simulink model "Watermarker"  (R2022a)
settings: Solver=FixedStepDiscrete  StartTime=0.0  StopTime=256*256-1  RelTol=1e-3
values from neighbouring files (symbols this model uses):
  alpha = 7    [example_set.mat]
  T0 = [1 1 1 0 0 0 0 0 1 1 1 0 ... (1024 elements, 1024x1)]    [example_set.mat]
  T1 = [1 1 0 0 0 0 0 0 0 0 0 1 ... (1024 elements, 1024x1)]    [example_set.mat]
libraries: hdlsllib x10, dspsrcs4 x4
Description:
  | Performs watermarking.
  | In:
  | - One channel of 8-bit image 256x256
  | - Watermark (64 bits)
  | Out:
  | - Watermarked image channel
settings Model: DataTypeOverride=Off  SimulationMode=accelerator  Creator=The MathWorks, Inc.  LastModifiedBy=Администратор
settings SolverCC: AlgebraicLoopSolver=TrustRegion
settings DataIOCC: LimitDataPoints=on  SaveFormat=Structure  SaveTime=off  ReturnWorkspaceOutputs=off
settings OptimizationCC: BlockReduction=off  ConditionallyExecuteInputs=off  DefaultParameterBehavior=Inlined  InheritOutputTypeSmallerThanSingle=on  LifeSpan=inf
settings DebuggingCC: AlgebraicLoopMsg=error  UnderspecifiedInitializationDetection=Classic  MergeDetectMultiDrivingBlocksExec=none  SolverPrmCheckMsg=warning  SingleTaskRateTransMsg=error  ParameterPrecisionLossMsg=none  UnconnectedInputMsg=warning  UnconnectedOutputMsg=warning  UnconnectedLineMsg=warning  AllowSymbolicDim=off  SFUnexpectedBacktrackingDiag=warning  SFNoUnconditionalDefaultTransitionDiag=warning  SFExecutionAtInitializationDiag=none  SFMachineParentedDataDiag=warning  ArithmeticOperatorsInVariantConditions=warning
settings HardwareCC: ProdBitPerPointer=32  ProdBitPerSizeT=32  ProdBitPerPtrDiffT=32  ProdLargestAtomicFloat=None  ProdIntDivRoundTo=Undefined  ProdEndianess=Unspecified  ProdWordSize=32  ProdHWDeviceType=ASIC/FPGA->ASIC/FPGA  TargetBitPerPointer=64  TargetBitPerSizeT=64  TargetBitPerPtrDiffT=64  TargetLongLongMode=on  TargetIntDivRoundTo=Zero  TargetEndianess=LittleEndian  TargetWordSize=64  TargetHWDeviceType=Custom Processor->MATLAB Host Computer  ProdEqTarget=off
settings ModelReferenceCC: PropagateSignalLabelsOutOfModel=off
settings SFSimCC: SimUseLocalCustomCode=off  CustomCodeUndefinedFunction=UseInterfaceOnly
settings RTWCC: RTWUseLocalCustomCode=off  DLArmComputeVersion=19.05
settings CodeAppCC: StateflowObjectComments=on
settings GRTTargetCC: TargetLangStandard=C89/C90 (ANSI)
settings ConfigComp: CovMetricSettings=dw  CovSaveCumulativeToWorkspaceVar=on  CovSaveSingleToWorkspaceVar=on  CovExternalEMLEnable=off  CovSFcnEnable=off

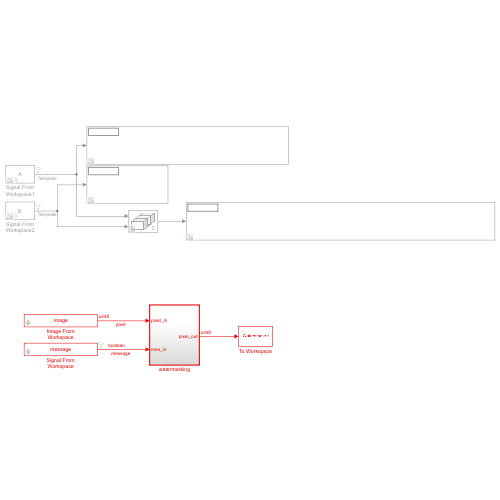
[thumbnail: Simulink's stored preview of the top-level diagram]
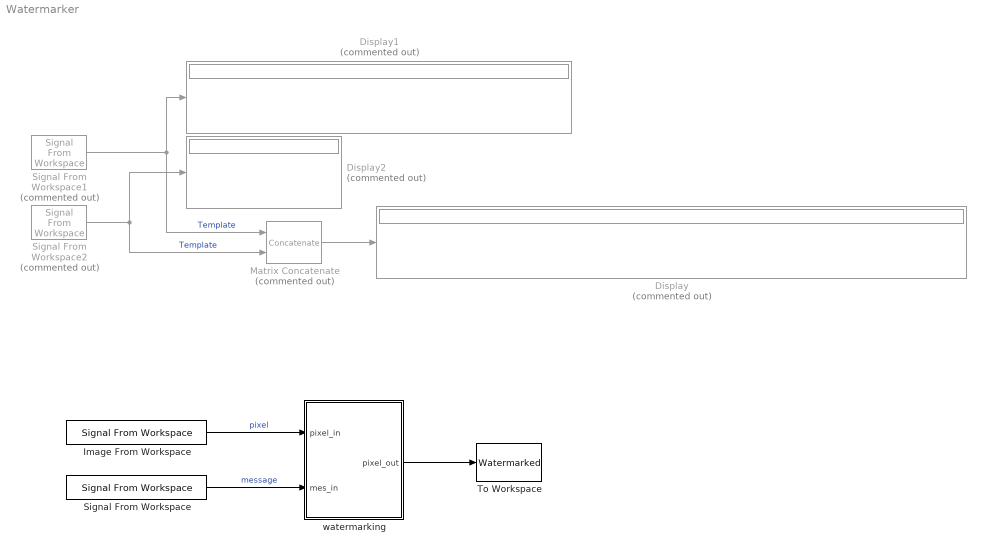
== system Watermarker ==
  Display : Display  Commented=on
      settings: Format=binary (Stored Integer)  Decimation=2
  Display1 : Display  Commented=on
      settings: Format=binary (Stored Integer)
  Display2 : Display  Commented=on
      settings: Format=binary (Stored Integer)
  Image From Workspace : dspsrcs4/Signal From Workspace  X=image  Ts=1  nsamps=1  OutputAfterFinalValue=Cyclic repetition  ignoreOrWarnInputAndFrameLengths=off  OutputFrames=off
  Matrix Concatenate : Concatenate  Commented=on  Mode=Multidimensional array  ConcatenateDimension=2
  Signal From Workspace : dspsrcs4/Signal From Workspace  X=message  Ts=1  nsamps=1  OutputAfterFinalValue=Cyclic repetition  ignoreOrWarnInputAndFrameLengths=off  OutputFrames=off
  Signal From Workspace1 : dspsrcs4/Signal From Workspace  Commented=on  X=A  Ts=1  nsamps=1  OutputAfterFinalValue=Cyclic repetition  ignoreOrWarnInputAndFrameLengths=off  OutputFrames=off
  Signal From Workspace2 : dspsrcs4/Signal From Workspace  Commented=on  X=B  Ts=1  nsamps=1  OutputAfterFinalValue=Cyclic repetition  ignoreOrWarnInputAndFrameLengths=off  OutputFrames=off
  To Workspace : ToWorkspace  VariableName=Watermarked  SampleTime=-1
      settings: Save2DSignal=2-D array (concatenate along first dimension)
  watermarking : Subsystem  TreatAsAtomicUnit=on
  wires:
  Image From Workspace/1 -> watermarking/1(pixel_in)  "pixel"
  Signal From Workspace/1 -> watermarking/2(mes_in)  "message"
  Signal From Workspace1/1 -> Display1/1, Matrix Concatenate/1  "Template"
  Signal From Workspace2/1 -> Matrix Concatenate/2, Display2/1  "Template"
  Matrix Concatenate/1 -> Display/1
  watermarking/1(pixel_out) -> To Workspace/1

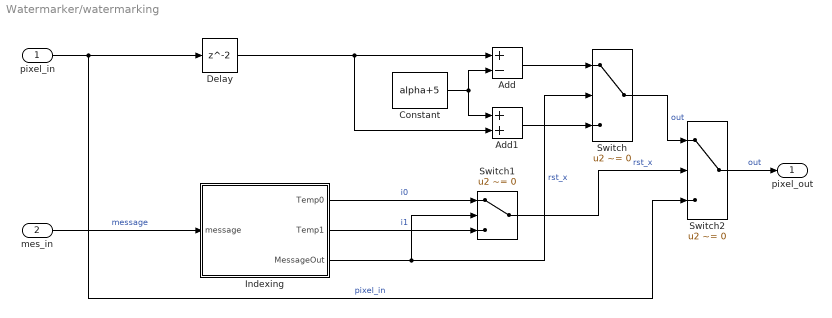
== system Watermarker/watermarking ==
  pixel_in : Inport
  mes_in : Inport  Port=2
  Add : Sum  Inputs=+-  OutMin=[0]  OutMax=[255]  OutDataTypeStr=uint8
  Add1 : Sum  OutMin=[0]  OutMax=[255]  OutDataTypeStr=uint8
  Constant : Constant  Value=alpha+5  SampleTime=-1
  Delay : Delay
  Indexing : Subsystem
  Switch : Switch  Criteria=u2 ~= 0  SaturateOnIntegerOverflow=off  InputSameDT=off
  Switch1 : Switch  Criteria=u2 ~= 0  SaturateOnIntegerOverflow=off  InputSameDT=off
  Switch2 : Switch  Criteria=u2 ~= 0  SaturateOnIntegerOverflow=off  InputSameDT=off
  pixel_out : Outport  VectorParamsAs1DForOutWhenUnconnected=off
  wires:
  mes_in/1 -> Indexing/1(message)  "message"
  Indexing/3(MessageOut) -> Switch1/2, Switch/2  "rst_x"
  pixel_in/1 -> Delay/1, Switch2/3  "pixel_in"
  Constant/1 -> Add1/1, Add/2
  Delay/1 -> Add1/2, Add/1
  Add/1 -> Switch/1
  Add1/1 -> Switch/3
  Switch/1 -> Switch2/1  "out"
  Indexing/1(Temp0) -> Switch1/1  "i0"
  Indexing/2(Temp1) -> Switch1/3  "i1"
  Switch1/1 -> Switch2/2  "rst_x"
  Switch2/1 -> pixel_out/1  "out"

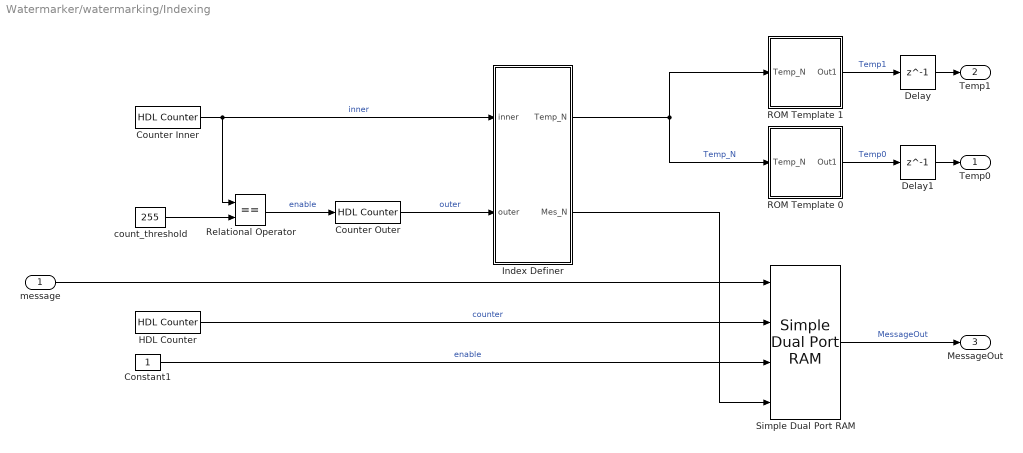
== system Watermarker/watermarking/Indexing ==
  message : Inport
  Constant1 : Constant  OutMin=[1]  OutMax=[1]  OutDataTypeStr=boolean  SampleTime=-1
  Counter Inner : hdlsllib/Sources/HDL Counter  CountType=Count limited  CountInit=0  CountStep=1  CountMax=255  CountFromType=Initial value  CountFrom=0  CountResetPort=off  CountLoadPort=off  CountEnbPort=off  CountDirPort=off  CountHitOutputPort=off  CountDataType=Unsigned  CountWordLen=8  CountFracLen=0  CountSampTime=1
  Counter Outer : hdlsllib/Sources/HDL Counter  CountType=Count limited  CountInit=0  CountStep=1  CountMax=255  CountFromType=Initial value  CountFrom=0  CountResetPort=off  CountLoadPort=off  CountEnbPort=on  CountDirPort=off  CountHitOutputPort=off  CountDataType=Unsigned  CountWordLen=8  CountFracLen=0  CountSampTime=1
  Delay : Delay  DelayLength=1  InitialCondition=0
  Delay1 : Delay  DelayLength=1  InitialCondition=0
  HDL Counter : hdlsllib/Sources/HDL Counter  CountType=Count limited  CountInit=0  CountStep=1  CountMax=63  CountFromType=Initial value  CountFrom=0  CountResetPort=off  CountLoadPort=off  CountEnbPort=off  CountDirPort=off  CountHitOutputPort=off  CountDataType=Unsigned  CountWordLen=6  CountFracLen=0  CountSampTime=1
  Index Definer : Subsystem
  ROM Template 0 : Subsystem
  ROM Template 1 : Subsystem
  Relational Operator : RelationalOperator  Operator===  OutDataTypeStr=boolean  InputSameDT=off
  Simple Dual Port RAM : hdlsllib/HDL RAMs/Simple Dual Port RAM  ram_size=6
      settings: SourceProductBaseCode=SL
  count_threshold : Constant  Value=255  OutMin=[255]  OutMax=[255]  OutDataTypeStr=uint8  SampleTime=-1
  Temp0 : Outport
  Temp1 : Outport  Port=2
  MessageOut : Outport  Port=3
  wires:
  HDL Counter/1 -> Simple Dual Port RAM/2  "counter"
  Counter Inner/1 -> Index Definer/1(inner), Relational Operator/1  "inner"
  count_threshold/1 -> Relational Operator/2
  Simple Dual Port RAM/1 -> MessageOut/1  "MessageOut"
  Relational Operator/1 -> Counter Outer/1  "enable"
  Constant1/1 -> Simple Dual Port RAM/3  "enable"
  Counter Outer/1 -> Index Definer/2(outer)  "outer"
  Index Definer/2(Mes_N) -> Simple Dual Port RAM/4
  Index Definer/1(Temp_N) -> ROM Template 0/1(Temp_N), ROM Template 1/1(Temp_N)  "Temp_N"
  ROM Template 0/1(Out1) -> Delay1/1  "Temp0"
  ROM Template 1/1(Out1) -> Delay/1  "Temp1"
  message/1 -> Simple Dual Port RAM/1
  Delay/1 -> Temp1/1
  Delay1/1 -> Temp0/1

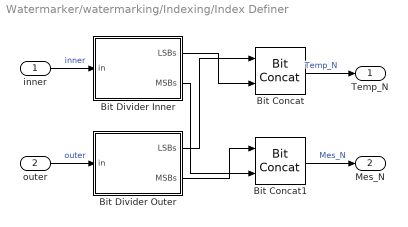
== system Watermarker/watermarking/Indexing/Index Definer ==
  inner : Inport
  outer : Inport  Port=2
  Bit Concat : hdlsllib/Logic and Bit Operations/Bit Concat  numInputs=2
  Bit Concat1 : hdlsllib/Logic and Bit Operations/Bit Concat  numInputs=2
  Bit Divider Inner : Subsystem
  Bit Divider Outer : Subsystem
  Temp_N : Outport
  Mes_N : Outport  Port=2
  wires:
  outer/1 -> Bit Divider Outer/1(in)  "outer"
  Bit Divider Inner/1(LSBs) -> Bit Concat/2
  Bit Concat/1 -> Temp_N/1  "Temp_N"
  Bit Concat1/1 -> Mes_N/1  "Mes_N"
  inner/1 -> Bit Divider Inner/1(in)  "inner"
  Bit Divider Outer/2(MSBs) -> Bit Concat1/1
  Bit Divider Inner/2(MSBs) -> Bit Concat1/2
  Bit Divider Outer/1(LSBs) -> Bit Concat/1

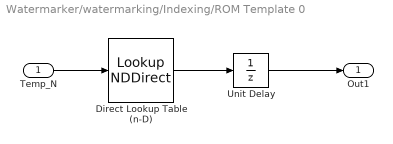
== system Watermarker/watermarking/Indexing/ROM Template 0 ==
  Temp_N : Inport
  Direct Lookup Table (n-D) : LookupNDDirect  NumberOfTableDimensions=1  Table=T0  DiagnosticForOutOfRangeInput=Error  TableMin=[0]  TableMax=[1]
  Unit Delay : UnitDelay  SampleTime=-1  HasFrameUpgradeWarning=on
  Out1 : Outport
  wires:
  Unit Delay/1 -> Out1/1
  Temp_N/1 -> Direct Lookup Table (n-D)/1
  Direct Lookup Table (n-D)/1 -> Unit Delay/1

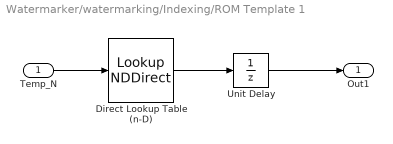
== system Watermarker/watermarking/Indexing/ROM Template 1 ==
  Temp_N : Inport
  Direct Lookup Table (n-D) : LookupNDDirect  NumberOfTableDimensions=1  Table=T1  DiagnosticForOutOfRangeInput=Error  TableMin=[0]  TableMax=[1]
  Unit Delay : UnitDelay  SampleTime=-1  HasFrameUpgradeWarning=on
  Out1 : Outport
  wires:
  Unit Delay/1 -> Out1/1
  Temp_N/1 -> Direct Lookup Table (n-D)/1
  Direct Lookup Table (n-D)/1 -> Unit Delay/1

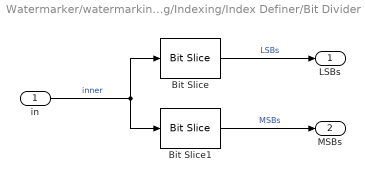
== system Watermarker/watermarking/Indexing/Index Definer/Bit Divider Inner ==
  in : Inport
  Bit Slice : hdlsllib/Logic and Bit Operations/Bit Slice  lidx=4  ridx=0
      settings: SourceProductBaseCode=SL
  Bit Slice1 : hdlsllib/Logic and Bit Operations/Bit Slice  lidx=7  ridx=5
      settings: SourceProductBaseCode=SL
  LSBs : Outport
  MSBs : Outport  Port=2
  wires:
  in/1 -> Bit Slice/1, Bit Slice1/1  "inner"
  Bit Slice/1 -> LSBs/1  "LSBs"
  Bit Slice1/1 -> MSBs/1  "MSBs"

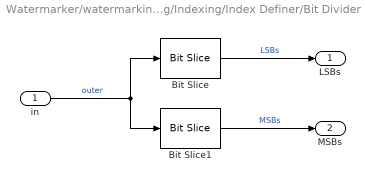
== system Watermarker/watermarking/Indexing/Index Definer/Bit Divider Outer ==
  in : Inport
  Bit Slice : hdlsllib/Logic and Bit Operations/Bit Slice  lidx=4  ridx=0
      settings: SourceProductBaseCode=SL
  Bit Slice1 : hdlsllib/Logic and Bit Operations/Bit Slice  lidx=7  ridx=5
      settings: SourceProductBaseCode=SL
  LSBs : Outport
  MSBs : Outport  Port=2
  wires:
  in/1 -> Bit Slice/1, Bit Slice1/1  "outer"
  Bit Slice/1 -> LSBs/1  "LSBs"
  Bit Slice1/1 -> MSBs/1  "MSBs"
